simulink model "IM_GA_model"  (R2014a)
settings: Solver=ode3  SolverMode=SingleTasking  StartTime=0.0  StopTime=100  FixedStep=Tsim  RelTol=1e-3
settings Model: Creator=3cap  LastModifiedBy=HC
settings DataIOCC: SignalLoggingSaveFormat=ModelDataLogs
settings OptimizationCC: ExpressionDepthLimit=2147483647  InitFltsAndDblsToZero=on
settings DebuggingCC: SaveWithParameterizedLinksMsg=none  UnderspecifiedInitializationDetection=Classic  SignalResolutionControl=TryResolveAllWithWarning  MultiTaskDSMMsg=warning  MultiTaskCondExecSysMsg=none  FcnCallInpInsideContextMsg=EnableAllAsWarning  StateNameClashWarn=warning
settings RTWCC: IncludeERTFirstTime=on
settings GRTTargetCC: TargetFcnLib=ansi_tfl_tmw.mat  CombineOutputUpdateFcns=off  GRTInterface=on

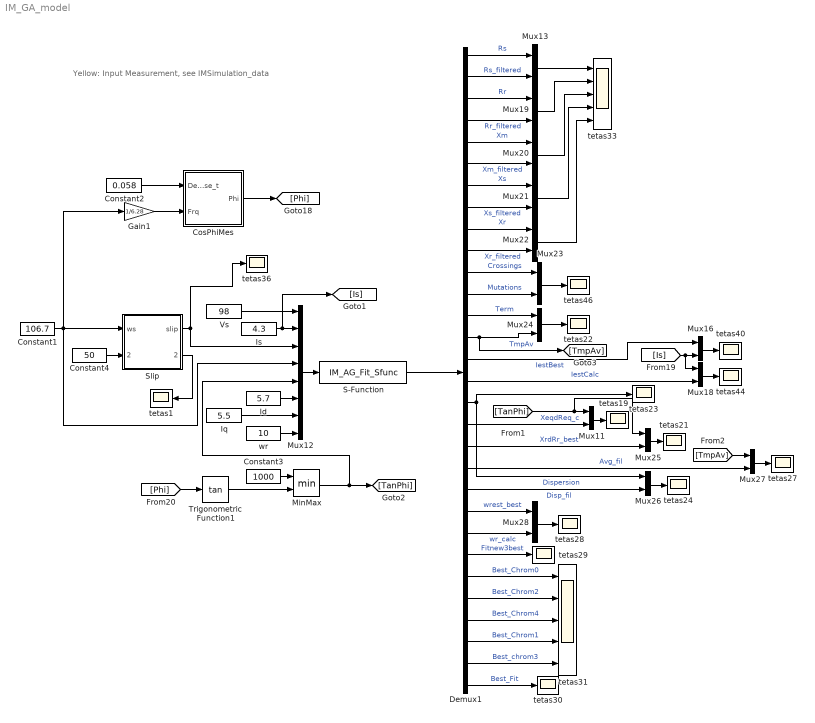
== system IM_GA_model ==
  note: Yellow: Input Measurement, see IMSimulation_data
  Constant1 : Constant  Value=106.7
  Constant2 : Constant  Value=0.058
  Constant3 : Constant  Value=1000
  Constant4 : Constant  Value=50
  CosPhiMes : Subsystem
  Demux1 : Demux  Outputs=30
  Gain1 : Gain  Gain=1/6.28
  Id : Constant  Value=5.7
  Iq : Constant  Value=5.5
  Is : Constant  Value=4.3
  MinMax : MinMax  Inputs=2
  Mux{11,13,16,18..28} (14 alike) : Mux  Inputs=2
  Mux12 : Mux  Inputs=8
  S-Function : S-Function  FunctionName=IM_AG_Fit_Sfunc  Parameters=Rs, Rr, Ls, Lr, Msr  EnableBusSupport=off
  Slip : Subsystem
  Trigonometric Function1 : Trigonometry  Operator=tan
  Vs : Constant  Value=98
  tetas{1,19,21..24,27..30,36,40,44,46} (14 alike) : Scope
      tetas1 settings: YMin=6.8  YMax=6.8  MaxDataPoints=5000000
      tetas19 settings: YMin=2.325  YMax=2.7  SaveName=ScopeData24  MaxDataPoints=5000000
      tetas21 settings: YMin=2  YMax=10  SaveName=ScopeData28  MaxDataPoints=5000000
      tetas22 settings: YMin=0  YMax=6.5  SaveName=ScopeData29  MaxDataPoints=5000000
      tetas23 settings: YMin=-45  YMax=45  SaveName=ScopeData30  MaxDataPoints=5000000
      tetas24 settings: YMin=0  YMax=25  SaveName=ScopeData31  MaxDataPoints=5000000
      tetas27 settings: YMin=0  YMax=4  SaveName=ScopeData32  MaxDataPoints=5000000
      tetas28 settings: YMin=0  YMax=3  SaveName=ScopeData33  MaxDataPoints=5000000
      tetas29 settings: YMin=0  YMax=150  SaveName=ScopeData47  MaxDataPoints=5000000
      tetas30 settings: YMin=0  YMax=150  SaveName=ScopeData49  MaxDataPoints=5000000
      tetas36 settings: YMin=0.109926  YMax=0.121498  SaveName=ScopeData37  MaxDataPoints=5000000
      tetas40 settings: YMin=1.25  YMax=4.5  SaveName=ScopeData40  MaxDataPoints=5000000
      tetas44 settings: YMin=9.43385  YMax=9.43485  SaveName=ScopeData45  MaxDataPoints=5000000
      tetas46 settings: YMin=145000  YMax=230000  SaveName=ScopeData48  MaxDataPoints=5000000
  tetas31 : Scope  NumInputPorts=5
      settings: YMin=1.78216~3.45611~4.50801~4.49715~4.41458  YMax=1.78216~3.45611~4.50801~4.49715~4.41458  SaveName=ScopeData50  MaxDataPoints=5000000
  tetas33 : Scope  NumInputPorts=5
      settings: YMin=5.618~2.1355~5.6375~5.6275~5.16  YMax=5.627~2.1395~5.655~5.645~5.1775  SaveName=ScopeData34  MaxDataPoints=5000000
  wr : Constant  Value=10
  wires:
  Mux12/1 -> S-Function/1
  S-Function/1 -> Demux1/1
  Is/1 -> [Is], Mux12/2
  Vs/1 -> Mux12/1
  Slip/1(slip) -> Mux12/3, tetas36/1
  Mux16/1 -> tetas40/1
  [Is] -> Mux18/1, Mux16/2
  Mux18/1 -> tetas44/1
  Demux1/1 -> Mux13/1  "Rs"
  Demux1/2 -> Mux13/2  "Rs_filtered"
  Mux13/1 -> tetas33/1
  Demux1/3 -> Mux19/1  "Rr"
  Demux1/4 -> Mux19/2  "Rr_filtered"
  Demux1/6 -> Mux20/2  "Xm_filtered"
  Mux20/1 -> tetas33/3
  Demux1/5 -> Mux20/1  "Xm"
  Demux1/7 -> Mux21/1  "Xs"
  Demux1/8 -> Mux21/2  "Xs_filtered"
  Mux21/1 -> tetas33/4
  Demux1/9 -> Mux22/1  "Xr"
  Demux1/10 -> Mux22/2  "Xr_filtered"
  Demux1/11 -> Mux23/1  "Crossings"
  Demux1/12 -> Mux23/2  "Mutations"
  Mux23/1 -> tetas46/1
  Demux1/15 -> Mux16/1  "IestBest"
  Demux1/16 -> Mux18/2  "IestCalc"
  Demux1/13 -> Mux24/1  "Term"
  Mux19/1 -> tetas33/2
  Mux22/1 -> tetas33/5
  CosPhiMes/1(Phi) -> [Phi]
  Mux11/1 -> tetas19/1
  [Phi] -> Trigonometric Function1/1
  Constant3/1 -> MinMax/1
  Constant1/1 -> Mux12/4, Slip/1(ws), Gain1/1
  Trigonometric Function1/1 -> MinMax/2
  Mux25/1 -> tetas21/1
  MinMax/1 -> [TanPhi], Mux12/5
  Demux1/19 -> Mux25/2  "XrdRr_best"
  Mux24/1 -> tetas22/1
  Demux1/14 -> [TmpAv], Mux24/2  "TmpAv"
  Demux1/17 -> tetas23/1, Mux26/1  "Dispersion"
  Mux26/1 -> tetas24/1
  Mux27/1 -> tetas27/1
  Demux1/20 -> Mux27/2  "Avg_fil"
  Demux1/21 -> Mux26/2  "Disp_fil"
  Slip/2(wr_mes) -> tetas1/1
  Id/1 -> Mux12/6
  Iq/1 -> Mux12/7
  wr/1 -> Mux12/8
  Mux28/1 -> tetas28/1
  Demux1/22 -> Mux28/1  "wrest_best"
  Demux1/23 -> Mux28/2  "wr_calc"
  Demux1/24 -> tetas29/1  "Fitnew3best"
  Demux1/26 -> tetas31/2  "Best_Chrom2"
  Demux1/27 -> tetas31/3  "Best_Chrom4"
  Demux1/25 -> tetas31/1  "Best_Chrom0"
  Demux1/28 -> tetas31/4  "Best_Chrom1"
  Demux1/29 -> tetas31/5  "Best_chrom3"
  Demux1/30 -> tetas30/1  "Best_Fit"
  Gain1/1 -> CosPhiMes/2("Frq ")
  Constant2/1 -> CosPhiMes/1(Dephase_t)
  Constant4/1 -> Slip/2(Speed)
  [TanPhi] -> Mux25/1, Mux11/1
  Demux1/18 -> Mux11/2  "XeqdReq_c"
  [TmpAv] -> Mux27/1

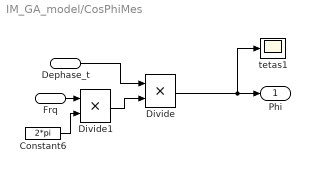
== system IM_GA_model/CosPhiMes ==
  Dephase_t : Inport
  "Frq " : Inport  Port=2
  Constant6 : Constant  Value=2*pi
  Divide : Product  Inputs=**
  Divide1 : Product  Inputs=**
  tetas1 : Scope
      settings: TimeRange=25  YMin=3.00752  YMax=3.00752  SaveName=ScopeData25  MaxDataPoints=5000000
  Phi : Outport
  wires:
  "Frq "/1 -> Divide1/1
  Constant6/1 -> Divide1/2
  Divide/1 -> tetas1/1, Phi/1
  Divide1/1 -> Divide/2
  Dephase_t/1 -> Divide/1

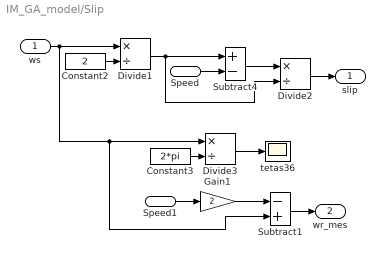
== system IM_GA_model/Slip ==
  ws : Inport
  Speed : Inport  Port=2
  Constant2 : Constant  Value=2
  Constant3 : Constant  Value=2*pi
  Divide1 : Product  Inputs=*/
  Divide2 : Product  Inputs=*/
  Divide3 : Product  Inputs=*/
  Gain1 : Gain  Gain=2
  Speed1 : InportShadow  Port=2
  Subtract1 : Sum  Inputs=-+
  Subtract4 : Sum  Inputs=+-
  tetas36 : Scope
      settings: YMin=0.135019  YMax=0.135023  SaveName=ScopeData44  MaxDataPoints=5000000
  slip : Outport
  wr_mes : Outport  Port=2
  wires:
  Constant2/1 -> Divide1/2
  Speed/1 -> Subtract4/2
  ws/1 -> Subtract1/2, Divide3/1, Divide1/1
  Divide1/1 -> Divide2/2, Subtract4/1
  Subtract4/1 -> Divide2/1
  Divide2/1 -> slip/1
  Constant3/1 -> Divide3/2
  Divide3/1 -> tetas36/1
  Subtract1/1 -> wr_mes/1
  Gain1/1 -> Subtract1/1
  Speed1/1 -> Gain1/1
